simulink model "project_7"  (R2019a)
settings: Solver=ode3  StartTime=0.0  StopTime=Sim_Time  FixedStep=0.01  RelTol=1e-3  EnableMultiTasking=on
values from neighbouring files (symbols this model uses):
  b = 3.5077E-6    (= 3.5077e-06)    [project_10_run.m]    (also in project_3.m = 0.3; project_4_run.m = 0.1; project_7_run.m = 10; project_8_run.m = 10)
  k = 10    [project_3.m]    (also in project_4_run.m = 20; project_7_run.m = 20; project_8_run.m = 20)
  Kd = 50    [project_7_run.m]    (also in project_8_run.m = 200)
  Ki = 300    [project_7_run.m]    (also in project_8_run.m = 200; project_9.m = 40)
  Kp = 350    [project_7_run.m]    (also in project_8_run.m = 300; project_9.m = 800)
  M = 1    [project_3.m]    (also in project_4_run.m; project_7_run.m; project_8_run.m)
  Step_Value = 1    [project_7_run.m]    (also in project_8_run.m)
settings Model: Creator=Nikita  LastModifiedBy=Nikita

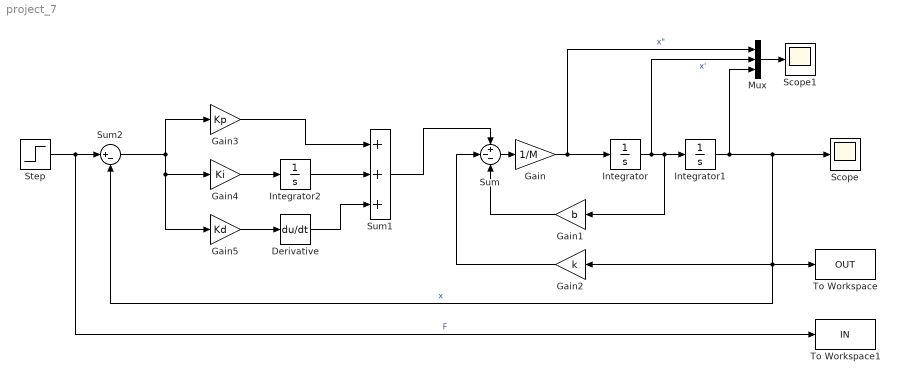
== system project_7 ==
  Derivative : Derivative
  Gain : Gain  Gain=1/M
  Gain1 : Gain  Gain=b
  Gain2 : Gain  Gain=k
  Gain3 : Gain  Gain=Kp
  Gain4 : Gain  Gain=Ki
  Gain5 : Gain  Gain=Kd
  Integrator : Integrator
  Integrator1 : Integrator
  Integrator2 : Integrator
  Mux : Mux  Inputs=3
  Scope : Scope
  Scope1 : Scope
  Step : Step  After=Step_Value  SampleTime=0
  Sum : Sum  Inputs=+--
  Sum1 : Sum  Inputs=+++
  Sum2 : Sum  Inputs=|+-
  To Workspace : ToWorkspace  VariableName=OUT  SaveFormat=Timeseries  SampleTime=-1
  To Workspace1 : ToWorkspace  VariableName=IN  SaveFormat=Timeseries  SampleTime=-1
  wires:
  Integrator1/1 -> Mux/3, Gain2/1, Sum2/2, To Workspace/1, Scope/1  "x"
  Gain1/1 -> Sum/3
  Gain/1 -> Mux/1, Integrator/1  "x\""
  Integrator2/1 -> Sum1/2
  Gain2/1 -> Sum/2
  Sum/1 -> Gain/1
  Gain3/1 -> Sum1/1
  Step/1 -> To Workspace1/1, Sum2/1  "F"
  Derivative/1 -> Sum1/3
  Integrator/1 -> Mux/2, Integrator1/1, Gain1/1  "x'"
  Gain4/1 -> Integrator2/1
  Sum2/1 -> Gain5/1, Gain4/1, Gain3/1
  Sum1/1 -> Sum/1
  Mux/1 -> Scope1/1
  Gain5/1 -> Derivative/1
